simulink model "Subsystem"  (R2020b)
settings: Solver=VariableStepAuto  StartTime=0.0  StopTime=10.0  RelTol=1e-3
settings Model: Creator=Yeshwanth  LastModifiedBy=Yeshwanth
settings DataIOCC: SaveOutput=off  SaveTime=off

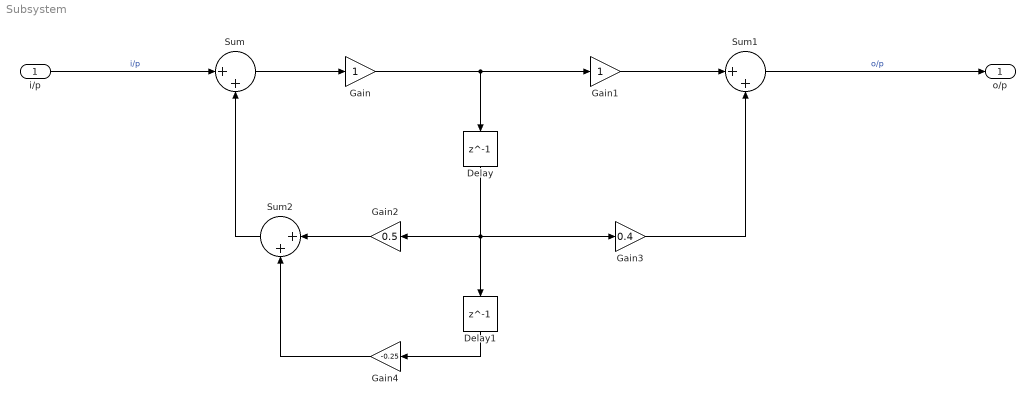
== system Subsystem ==
  i/p : Inport  OutDataTypeStr=double  PortDimensions=1  SampleTime=0
  Delay : Delay  DelayLength=1
  Delay1 : Delay  DelayLength=1
  Gain : Gain
  Gain1 : Gain
  Gain2 : Gain  Gain=0.5
  Gain3 : Gain  Gain=0.4
  Gain4 : Gain  Gain=-0.25
  Sum : Sum  Inputs=|++
  Sum1 : Sum  Inputs=|++
  Sum2 : Sum  Inputs=|++
  o/p : Outport  OutDataTypeStr=double  PortDimensions=1  SampleTime=0
  wires:
  Gain3/1 -> Sum1/2
  Gain/1 -> Gain1/1, Delay/1
  Sum2/1 -> Sum/2
  Sum/1 -> Gain/1
  Delay1/1 -> Gain4/1
  Delay/1 -> Delay1/1, Gain2/1, Gain3/1
  Gain1/1 -> Sum1/1
  Gain4/1 -> Sum2/2
  Gain2/1 -> Sum2/1
  i/p/1 -> Sum/1  "i/p"
  Sum1/1 -> o/p/1  "o/p"
